simulink model "with_acceleration"  (R2021a)
settings: Solver=VariableStepAuto  StartTime=0.0  StopTime=10.0  RelTol=1e-3
settings Model: Creator=Osman  LastModifiedBy=Osman

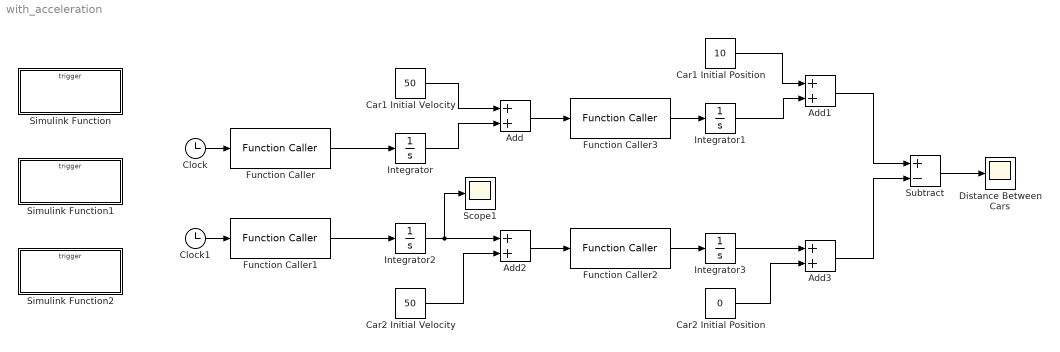
== system with_acceleration ==
  Add : Sum
  Add1 : Sum
  Add2 : Sum  OutDataTypeStr=double
  Add3 : Sum  OutDataTypeStr=double
  Car1 Initial Position : Constant  Value=10
  Car1 Initial Velocity : Constant  Value=50
  Car2 Initial Position : Constant  Value=0
  Car2 Initial Velocity : Constant  Value=50
  Clock : Clock
  Clock1 : Clock
  Distance Between Cars : Scope
  Function Caller : FunctionCaller  FunctionPrototype=y = acc1(u)  InputArgumentSpecifications=<Enter example>  OutputArgumentSpecifications=<Enter example>
  Function Caller1 : FunctionCaller  FunctionPrototype=y = acc2(u)  InputArgumentSpecifications=<Enter example>  OutputArgumentSpecifications=<Enter example>
  Function Caller2 : FunctionCaller  FunctionPrototype=y = vel_conv(u)  InputArgumentSpecifications=<Enter example>  OutputArgumentSpecifications=<Enter example>
  Function Caller3 : FunctionCaller  FunctionPrototype=y = vel_conv(u)  InputArgumentSpecifications=<Enter example>  OutputArgumentSpecifications=<Enter example>
  Integrator{,1..3} (4 alike) : Integrator
  Scope1 : Scope
  Simulink Function : Subsystem  TreatAsAtomicUnit=on
  Simulink Function1 : Subsystem  TreatAsAtomicUnit=on
  Simulink Function2 : Subsystem  TreatAsAtomicUnit=on
  Subtract : Sum  Inputs=+-  OutDataTypeStr=double
  wires:
  Clock/1 -> Function Caller/1
  Function Caller/1 -> Integrator/1
  Car1 Initial Velocity/1 -> Add/1
  Integrator/1 -> Add/2
  Car1 Initial Position/1 -> Add1/1
  Integrator1/1 -> Add1/2
  Clock1/1 -> Function Caller1/1
  Function Caller1/1 -> Integrator2/1
  Integrator2/1 -> Scope1/1, Add2/1
  Car2 Initial Velocity/1 -> Add2/2
  Integrator3/1 -> Add3/1
  Car2 Initial Position/1 -> Add3/2
  Add1/1 -> Subtract/1
  Add3/1 -> Subtract/2
  Subtract/1 -> Distance Between Cars/1
  Add/1 -> Function Caller3/1
  Function Caller2/1 -> Integrator3/1
  Add2/1 -> Function Caller2/1
  Function Caller3/1 -> Integrator1/1

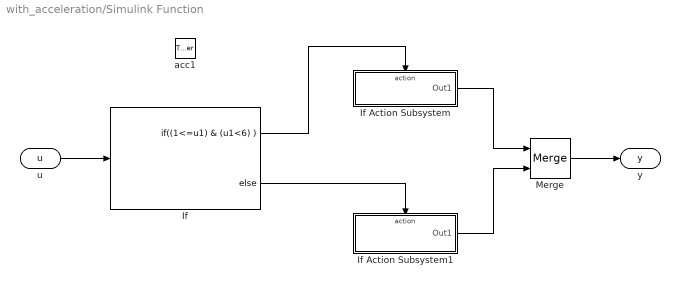
== system with_acceleration/Simulink Function ==
  acc1 : TriggerPort  TriggerType=function-call  IsSimulinkFunction=on  FunctionName=acc1  FunctionVisibility=scoped  VariantControl=(inherit)
  If : If  IfExpression=(1<=u1) & (u1<6)
  If Action Subsystem : Subsystem  TreatAsAtomicUnit=on
  If Action Subsystem1 : Subsystem  TreatAsAtomicUnit=on
  Merge : Merge
  u : ArgIn  DisableCoverage=on  ArgumentName=u
  y : ArgOut  DisableCoverage=on  ArgumentName=y
  wires:
  If/1 -> If Action Subsystem/Action
  If Action Subsystem/1(Out1) -> Merge/1
  If Action Subsystem1/1(Out1) -> Merge/2
  If/2 -> If Action Subsystem1/Action
  u/1 -> If/1
  Merge/1 -> y/1

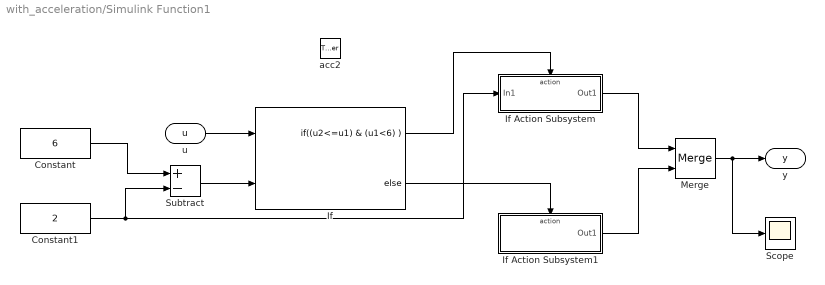
== system with_acceleration/Simulink Function1 ==
  acc2 : TriggerPort  TriggerType=function-call  IsSimulinkFunction=on  FunctionName=acc2  FunctionVisibility=scoped  VariantControl=(inherit)
  Constant : Constant  Value=6
  Constant1 : Constant  Value=2  OutDataTypeStr=double  LockScale=on
  If : If  NumInputs=2  IfExpression=(u2<=u1) & (u1<6)
  If Action Subsystem : Subsystem  TreatAsAtomicUnit=on
  If Action Subsystem1 : Subsystem  TreatAsAtomicUnit=on
  Merge : Merge
  Scope : Scope
  Subtract : Sum  Inputs=+-  OutDataTypeStr=double  RndMeth=Convergent
  u : ArgIn  DisableCoverage=on  ArgumentName=u
  y : ArgOut  DisableCoverage=on  ArgumentName=y
  wires:
  If/1 -> If Action Subsystem/Action
  If Action Subsystem/1(Out1) -> Merge/1
  If Action Subsystem1/1(Out1) -> Merge/2
  If/2 -> If Action Subsystem1/Action
  u/1 -> If/1
  Merge/1 -> Scope/1, y/1
  Constant/1 -> Subtract/1
  Constant1/1 -> If Action Subsystem/1(In1), Subtract/2
  Subtract/1 -> If/2

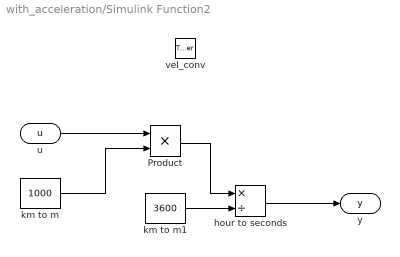
== system with_acceleration/Simulink Function2 ==
  vel_conv : TriggerPort  TriggerType=function-call  IsSimulinkFunction=on  FunctionName=vel_conv  FunctionVisibility=scoped  VariantControl=(inherit)
  Product : Product
  hour to seconds : Product  Inputs=*/
  km to m : Constant  Value=1000
  km to m1 : Constant  Value=3600
  u : ArgIn  DisableCoverage=on  ArgumentName=u
  y : ArgOut  DisableCoverage=on  ArgumentName=y
  wires:
  u/1 -> Product/1
  km to m/1 -> Product/2
  km to m1/1 -> hour to seconds/2
  Product/1 -> hour to seconds/1
  hour to seconds/1 -> y/1

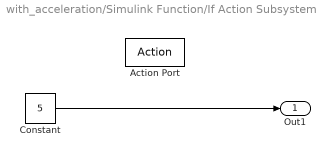
== system with_acceleration/Simulink Function/If Action Subsystem ==
  Action Port : ActionPort  ActionPortLabel=if((1<=u1) & (u1<6) )
  Constant : Constant  Value=5
  Out1 : Outport
  wires:
  Constant/1 -> Out1/1

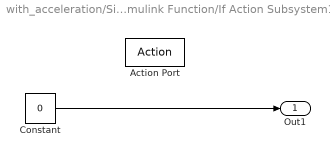
== system with_acceleration/Simulink Function/If Action Subsystem1 ==
  Action Port : ActionPort  ActionPortLabel=else
  Constant : Constant  Value=0
  Out1 : Outport
  wires:
  Constant/1 -> Out1/1

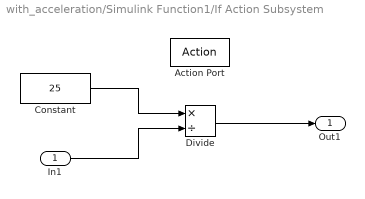
== system with_acceleration/Simulink Function1/If Action Subsystem ==
  In1 : Inport
  Action Port : ActionPort  ActionPortLabel=if((u2<=u1) & (u1<6) )
  Constant : Constant  Value=25
  Divide : Product  Inputs=*/  OutDataTypeStr=double
  Out1 : Outport
  wires:
  Divide/1 -> Out1/1
  Constant/1 -> Divide/1
  In1/1 -> Divide/2

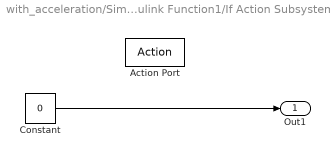
== system with_acceleration/Simulink Function1/If Action Subsystem1 ==
  Action Port : ActionPort  ActionPortLabel=else
  Constant : Constant  Value=0
  Out1 : Outport
  wires:
  Constant/1 -> Out1/1
